simulink model "simulation"  (Simulink 9.2)
settings: Solver=FixedStepAuto  StartTime=0.0  StopTime=50  RelTol=1e-3  EnableMultiTasking=on
PreLoadFcn:
  | % Motor Parameters
  | 
  | J=0.01;     %kg*m^2
  | b=0.1;      %N*m/(rad/s)
  | K=0.01;     %V/(rad/s)
  | R=1;        %Ohm
  | L=0.5;      %H
libraries: simulink x1, embdlinuxlib x1, raspberrypilib x1
settings Model: Creator=deastman  LastModifiedBy=computer  SimulationMode=external  ExtModeBatchMode=on
settings SolverCC: ConcurrentTasks=on  PositivePriorityOrder=on  AutoInsertRateTranBlk=on
settings OptimizationCC: EnhancedBackFolding=on  PassReuseOutputArgsAs=Individual arguments  ExpressionDepthLimit=2147483647  InitFltsAndDblsToZero=on  LifeSpan=auto  MaxStackSize=64  OptimizeBlockOrder=speed  DifferentSizesBufferReuse=on  OptimizationCustomize=off
settings DebuggingCC: SolverPrmCheckMsg=warning  ParameterTunabilityLossMsg=error
settings HardwareCC: ProdLargestAtomicInteger=Long  ProdLargestAtomicFloat=Double  ProdIntDivRoundTo=Zero  ProdEndianess=LittleEndian  ProdHWDeviceType=ARM Compatible->ARM Cortex  UseEmbeddedCoderFeatures=off  UseSimulinkCoderFeatures=off
settings SFSimCC: MATLABDynamicMemAlloc=off
settings RTWCC: SystemTargetFile=ert.tlc  HardwareBoard=Raspberry Pi  TLCOptions="-aInlineSetEventsForThisBaseRateFcn=TLC_FALSE -aSuppressMultiTaskScheduler=TLC_FALSE  -aRateBasedStepFcn=0"  TemplateMakefile=ert_default_tmf  Description=Embedded Coder  GenerateReport=on  Toolchain=GNU GCC Raspberry Pi  BuildConfiguration=Faster Runs  IncludeHyperlinkInReport=on  LaunchReport=on  GenerateTraceInfo=on  GenerateTraceReport=on  GenerateTraceReportSl=on  GenerateTraceReportSf=on  GenerateTraceReportEml=on
settings MATStruct: className=codertarget.tools.BuildHook  argsTopModelOnly=[]  excludedModels=[]  includeReferencedModels=on  includeTopModel=on  enabled=on  UseCoderTarget=[1.0]  TargetHardware=Raspberry Pi  RTOS=Linux  RTOSBaseRateTaskPriority=40  DetectTaskOverruns=[1.0]  Scheduler_interrupt_source=[0.0]  DataVersion=2016.02  IPAddress=codertarget.raspi.getDeviceAddress  Port=17725  Verbose=[0.0]  RunInBackground=[0.0]  Configuration=TCP/IP  DeviceAddress=10.66.223.107  Username=pi  Password=DeepPiCar  BuildDir=/home/pi/cps  BuildAction=Build and run  RunOnBoot=[0.0]  SPI0CE0BusSpeed=500  SPI0CE1BusSpeed=500  BrokerAddress=mqtt.thingspeak.com
settings CodeAppCC: ForceParamTrailComments=on  IgnoreCustomStorageClasses=off  OperatorAnnotations=on  SimulinkDataObjDesc=on  SFDataObjDesc=on  MangleLength=10  InsertBlockDesc=on  StateflowObjectComments=off
settings ERTTargetCC: SupportNonInlinedSFcns=on  SupportVariableSizeSignals=on

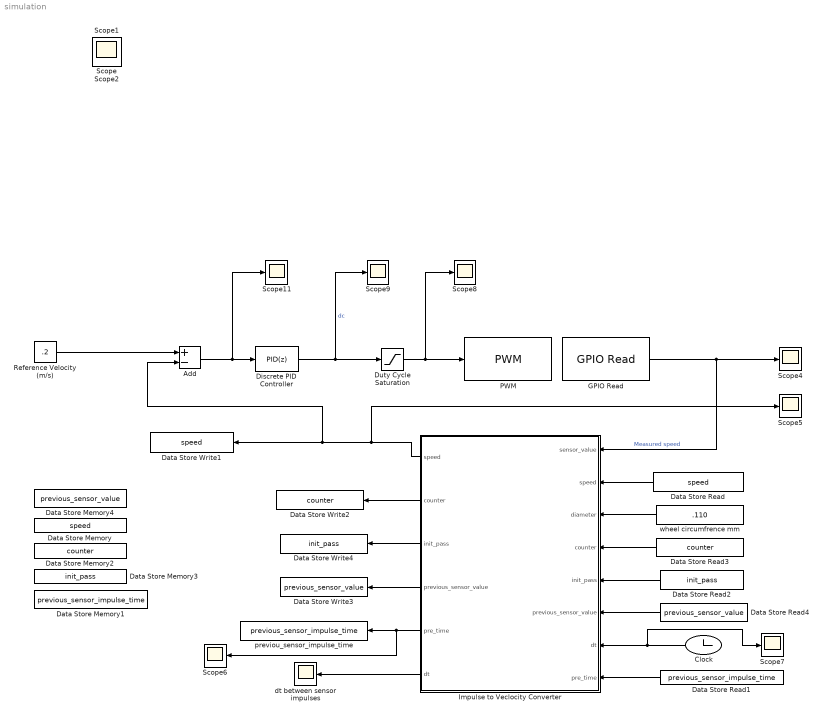
== system simulation ==
  Add : Sum  Inputs=+-
  "Clock " : Clock
  Data Store Memory : DataStoreMemory  DataStoreName=speed  ReadBeforeWriteMsg=warning  WriteAfterWriteMsg=warning  WriteAfterReadMsg=warning  ShowAdditionalParam=off
  Data Store Memory1 : DataStoreMemory  DataStoreName=previous_sensor_impulse_time  ReadBeforeWriteMsg=warning  WriteAfterWriteMsg=warning  WriteAfterReadMsg=warning  ShowAdditionalParam=off
  Data Store Memory2 : DataStoreMemory  DataStoreName=counter  ReadBeforeWriteMsg=warning  WriteAfterWriteMsg=warning  WriteAfterReadMsg=warning  ShowAdditionalParam=off
  Data Store Memory3 : DataStoreMemory  DataStoreName=init_pass  ReadBeforeWriteMsg=warning  WriteAfterWriteMsg=warning  WriteAfterReadMsg=warning  ShowAdditionalParam=off
  Data Store Memory4 : DataStoreMemory  DataStoreName=previous_sensor_value  ReadBeforeWriteMsg=warning  WriteAfterWriteMsg=warning  WriteAfterReadMsg=warning  ShowAdditionalParam=off
  Data Store Read : DataStoreRead  DataStoreName=speed
  Data Store Read1 : DataStoreRead  DataStoreName=previous_sensor_impulse_time
  Data Store Read2 : DataStoreRead  DataStoreName=init_pass
  Data Store Read3 : DataStoreRead  DataStoreName=counter
  Data Store Read4 : DataStoreRead  DataStoreName=previous_sensor_value
  Data Store Write1 : DataStoreWrite  DataStoreName=speed
  Data Store Write2 : DataStoreWrite  DataStoreName=counter
  Data Store Write3 : DataStoreWrite  DataStoreName=previous_sensor_value
  Data Store Write4 : DataStoreWrite  DataStoreName=init_pass
  Discrete PID Controller : simulink/Continuous/PID Controller  Controller=PID  Form=Parallel  TimeDomain=Discrete-time  SampleTime=0.001  IntegratorMethod=Forward Euler  FilterMethod=Forward Euler  ControllerParametersSource=internal  P=.013  I=.0001  D=.0002  UseFilter=on  N=160.6  TunerSelectOption=Transfer Function Based (PID Tuner App)  InitialConditionSource=internal  InitialConditionForIntegrator=0  InitialConditionForFilter=0  DifferentiatorICPrevScaledInput=0  ExternalReset=none  TrackingMode=off  Kt=1  LimitOutput=off  UpperSaturationLimit=10  LowerSaturationLimit=-10  LinearizeAsGain=on  AntiWindupMode=back-calculation  Kb=1  POutMin=[]  POutMax=[]  IOutMin=[]  IOutMax=[]  DOutMin=[]  DOutMax=[]  NOutMin=[]  NOutMax=[]  SumOutMin=[]  SumOutMax=[]  SaturationOutMin=[]  SaturationOutMax=[]  PParamMin=[]  PParamMax=[]  IParamMin=[]  IParamMax=[]  DParamMin=[]  DParamMax=[]  NParamMin=[]  NParamMax=[]  KbParamMin=[]  KbParamMax=[]  KtParamMin=[]  KtParamMax=[]  KbOutMin=[]  KbOutMax=[]  KtOutMin=[]  KtOutMax=[]  IntegratorOutMin=[]  IntegratorOutMax=[]  FilterOutMin=[]  FilterOutMax=[]  SumI1OutMin=[]  SumI1OutMax=[]  SumI2OutMin=[]  SumI2OutMax=[]  SumI3OutMin=[]  SumI3OutMax=[]  SumI4OutMin=[]  SumI4OutMax=[]  SumDOutMin=[]  SumDOutMax=[]  DifferentiatorOutMin=[]  DifferentiatorOutMax=[]  FilterDiffOutCoefMin=[]  FilterDiffOutCoefMax=[]  ReciprocalOutMin=[]  ReciprocalOutMax=[]  SumDenOutMin=[]  SumDenOutMax=[]  SumNumOutMin=[]  SumNumOutMax=[]  DivideOutMin=[]  DivideOutMax=[]  IntegratorContinuousStateAttributes=''  IntegratorStateMustResolveToSignalObject=off  IntegratorRTWStateStorageClass=Auto  FilterContinuousStateAttributes=''  FilterStateMustResolveToSignalObject=off  FilterRTWStateStorageClass=Auto  ParallelPVariant=InternalParameters  IdealPVariant=Disabled  IVariant=InternalParameters  DVariant=InternalParameters  IntegratorVariant=Discrete  SatVariant=Disabled  AWVariant=Passthrough  PCopyVariant=Disabled  TRVariant=Disabled  FdbkBlocksVariant=Forward  IdealPFdbkVariant=Disabled  SatFdbkVariant=Disabled  DerivativeFilterVariant=ForwardEulerFilter  NVariant=InternalParameters  NCopyVariant=Disabled  FilterICVariant=InternalICsFilter  IntegratorICVariant=InternalICs  ExternalResetVariant=Disabled  TRSumVariant=Passthrough  SumFdbkVariant=Disabled  SumVariant=Sum_PID
  Duty Cycle Saturation : Saturate  UpperLimit=.162  LowerLimit=.158
  GPIO Read : embdlinuxlib/GPIO Read  board=Pi 3 Model B  gpio=21  internalResistor=Off  sampleTime=.01  direction=Input  blockPlatform=Raspberry Pi
      settings: SourceProductName=Simulink Support Package for Raspberry Pi Hardware  SourceProductBaseCode=RASPPI
  Impulse to Veclocity Converter : MATLAB Function  TreatAsAtomicUnit=on
  PWM : raspberrypilib/PWM  board=Pi 3 Model B  Pin_=18  Frequency=100  blockPlatform=Raspberry Pi
      settings: SourceProductName=Simulink Support Package for Raspberry Pi Hardware  SourceProductBaseCode=RASPPI
  Reference Velocity (m/s) : Constant  Value=.2  SampleTime=-1
  Scope{,1..2,4..9,11} (10 alike) : Scope
  dt between sensor impulses : Scope
  previou_sensor_impulse_time : DataStoreWrite  DataStoreName=previous_sensor_impulse_time
  wheel circumfrence mm : Constant  Value=.110  SampleTime=-1
  wires:
  GPIO Read/1 -> Impulse to Veclocity Converter/1(sensor_value), Scope4/1  "Measured speed"
  Discrete PID Controller/1 -> Scope9/1, Duty Cycle Saturation/1  "dc"
  Reference Velocity (m/s)/1 -> Add/1
  wheel circumfrence mm/1 -> Impulse to Veclocity Converter/3(diameter)
  Data Store Read/1 -> Impulse to Veclocity Converter/2("speed ")
  Impulse to Veclocity Converter/1(speed) -> Scope5/1, Data Store Write1/1, Add/2
  Data Store Read3/1 -> Impulse to Veclocity Converter/4("counter ")
  Impulse to Veclocity Converter/2(counter) -> Data Store Write2/1
  Impulse to Veclocity Converter/3(init_pass) -> Data Store Write4/1
  Data Store Read2/1 -> Impulse to Veclocity Converter/5("init_pass ")
  Data Store Read4/1 -> Impulse to Veclocity Converter/6("previous_sensor_value ")
  Impulse to Veclocity Converter/4(previous_sensor_value) -> Data Store Write3/1
  "Clock "/1 -> Impulse to Veclocity Converter/7("dt "), Scope7/1
  Data Store Read1/1 -> Impulse to Veclocity Converter/8("pre_time ")
  Impulse to Veclocity Converter/5(pre_time) -> Scope6/1, previou_sensor_impulse_time/1
  Add/1 -> Scope11/1, Discrete PID Controller/1
  Duty Cycle Saturation/1 -> Scope8/1, PWM/1
  Impulse to Veclocity Converter/6(dt) -> dt between sensor impulses/1

== matlab function Impulse to Veclocity Converter ==
  data: sensor_value input double; speed output double; speed input double; diameter input double; counter input double; counter output double; init_pass output double; init_pass input double; previous_sensor_value output double; previous_sensor_value input double; dt input double; pre_time input double; pre_time output double; dt output double
function [speed, counter, init_pass, previous_sensor_value,pre_time, dt] = fcn(sensor_value, speed, diameter, counter, init_pass, previous_sensor_value, dt, pre_time)

counter = counter + 1;

%update time if not first sample
if(sensor_value == 1 && previous_sensor_value == 0 && init_pass == 1)
    dt = dt-pre_time;
    circum = diameter*pi;
    rps = (1 / dt);
    speed = rps*circum;
    counter = 0;
    pre_time = dt;
elseif(sensor_value == 1 && init_pass == 0)
    pre_time = dt;
    counter = 0;
    init_pass = 1;
end
